simulink model "VL53L0X"  (R2017b)
settings: Solver=FixedStepDiscrete  StartTime=0.0  StopTime=10.0  FixedStep=1e-3  RelTol=1e-3
libraries: mbed_lib x4, mbed_i2c_sensors x1
settings Model: Creator=oh  LastModifiedBy=oh
settings DataIOCC: LimitDataPoints=on  SaveFormat=Array
settings OptimizationCC: DefaultParameterBehavior=Inlined  PassReuseOutputArgsAs=Individual arguments
settings DebuggingCC: ParameterTunabilityLossMsg=error  SFUnexpectedBacktrackingDiag=warning  SFNoUnconditionalDefaultTransitionDiag=warning  SFExecutionAtInitializationDiag=none
settings HardwareCC: ProdBitPerPointer=32  ProdBitPerSizeT=32  ProdBitPerPtrDiffT=32  ProdLargestAtomicInteger=Long  ProdLargestAtomicFloat=Double  ProdWordSize=32  ProdHWDeviceType=ARM Compatible->ARM Cortex
settings ModelReferenceCC: PropagateSignalLabelsOutOfModel=off
settings SFSimCC: MATLABDynamicMemAlloc=off
settings RTWCC: SystemTargetFile=mbed.tlc  TemplateMakefile=mbed.tmf  Description=MbedTarget (Embedded Target for Embedded Coder)  IncludeHyperlinkInReport=on  TargetLang=C++
settings CodeAppCC: ForceParamTrailComments=on  IgnoreCustomStorageClasses=off  OperatorAnnotations=on  SimulinkDataObjDesc=on  SFDataObjDesc=on  InsertBlockDesc=on
settings STFCustomTargetCC: TargetLibSuffix=.a  MultiwordLength=256  GenerateSampleERTMain=on  CombineOutputUpdateFcns=on  ERTCustomFileBanners=on  SupportContinuousTime=off  SupportNonInlinedSFcns=off  RemoveResetFunc=on  MATLABClassNameForMDSCustomization=Simulink.SoftwareTarget.ERTCustomization  ModelStepFunctionPrototypeControlCompliant=on  GRTInterface=off  SystemTargetFile=mbed.tlc
settings ERTTargetCC: GenerateSampleERTMain=on  ParMdlRefBuildCompliant=off  CompOptLevelCompliant=off  ConcurrentExecutionCompliant=off  CPPClassGenCompliant=off  UseToolchainInfoCompliant=off  InlinedParameterPlacement=NonHierarchical  ERTCustomFileTemplate=mbed_file_process.tlc
settings ConfigComp: CovMetricSettings=dw  CovHtmlReporting=on  CovSaveCumulativeToWorkspaceVar=on  CovSaveSingleToWorkspaceVar=on  CovExternalEMLEnable=off

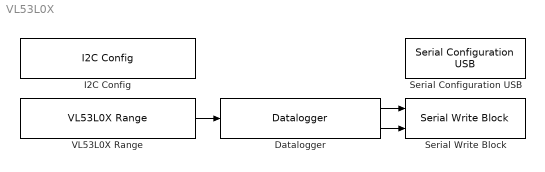
== system VL53L0X ==
  Datalogger : mbed_lib/Utilities/Datalogger  TypeInputPorts={ 'uint16' 1 }  TypeOfInputs={'1*uint16'}  BufferSize=100  errEn=off  SampleTime=-1
      settings: SourceProductName=Mbed Target
  I2C Config : mbed_lib/Serial/I2C/I2C Config  Priority=0  I2CPort=1  Freq=100000  SDAPortName=B  SDAPinNumber=9  SCLPortName=B  SCLPinNumber=8
      settings: SourceProductName=Mbed Target
  Serial Configuration USB : mbed_lib/Serial/UART/Serial Configuration USB  BaudRate=9600
      settings: SourceProductName=Mbed Target
  Serial Write Block : mbed_lib/Serial/UART/Serial Write Block  SerialPort=USB  numData=on  SampleTime=-1
      settings: SourceProductName=Mbed Target
  VL53L0X Range : mbed_i2c_sensors/VL53L0X Range  i2cbus=1  Mode=single polling  IntPortName=A  IntPinNumber=4  ShutPortName=C  ShutPinNumber=6  EnableError=off  SampleTime=-1
      settings: SourceProductName=Mbed Target
  wires:
  VL53L0X Range/1 -> Datalogger/1
  Datalogger/1 -> Serial Write Block/1
  Datalogger/2 -> Serial Write Block/2
